simulink model "VDCHyd2022a"  (R2022a)
settings: Solver=daessc  StartTime=0.0  StopTime=simulationEndTime  FixedStep=0.001  RelTol=1e-2
values from neighbouring files (symbols this model uses):
  aux = thetaXrLB(i)    [initInertiaUpdate.m]
  Bc1_V = [0;0;0;0;0;0]    [InitializeSimulationParameters.m]
  Bc1_Vr = [0;0;0;0;0;0]    [InitializeSimulationParameters.m]
  D22Fr = [0;0;0;0;0;0]    [InitializeSimulationParameters.m]
  filtDF = init2ndOrderLowPassFilter(filtDF.cutOffFrequency,1,controller.dT)    [initializeLowPassFilters.m]
  filtDV = init2ndOrderLowPassFilter(filtDV.cutOffFrequency,1,controller.dT)    [initializeLowPassFilters.m]
  filtEnc = init2ndOrderLowPassFilter(filtEnc.cutOffFrequency,1,controller.dT)    [initializeLowPassFilters.m]
  filtPres = init2ndOrderLowPassFilter(filtPres.cutOffFrequency,1,controller.dT)    [initializeLowPassFilters.m]
  MODE = 1    [RUN_ME.m]
  s = tf('s')    [init2ndOrderLowPassFilter.m]
undefined symbols (not defined in the file or in its folder): B11_r_B11Tc1, B11_V, B11_Vr, B11Ftot_r, B12_r_B12Tc2, B12_Rot_Tc2, B12_U_Tc2, B12_V, B12_Vr, B12Ftot_r, B31_r_B31B41, B31_V, B31_Vr, B31FTot_r, B32_r_B32B42, B32_Rot_B42, B32_U_B42, B32_V, B32_Vr, B32FTot_r, B41_r_B41Tc1, B41_V, B41_Vr, B41FTot_r, B42_r_B42Tc2, B42_Rot_Tc2, B42_U_Tc2, B42_V, B42_Vr, B42FTot_r, B52_r_B52P32, B52_Rot_P32, B52_U_P32, B52_V, B52_Vr, B52Ftot_r, Bc1_r_Bc1B11, Bc1_r_Bc1B31, Bc1FTot_r, Bc2_r_Bc2B12, Bc2_r_Bc2B32, Bc2_Rot_B12, Bc2_Rot_B32, Bc2_U_B12, Bc2_U_B32, Bc2_V, Bc2_Vr, Bc2Tot_r, controller, cyl1, cyl2, cylT2, D22_V, D22_Vr, DiscIntNeverNeededParam, dq1, dq11, dq11r, dq12, dq12r ... (+119)
libraries: sm_lib x34, nesl_utility x15, simulink x11, dspinverses x1
(part 11 of 12)

== matlab function VDCHyd2022a/sbVDCController/sbFormTotalRequiredForces/sbTotalRequiredForcesPS2/regressorYB52r ==
  data: B52Vr input; B52dVr input; B52V input; B52_Rot_W input; gravity parameter; YB52r output
function YB52r  = inertiaRegressor(B52Vr, B52dVr, B52V, B52_Rot_W,  gravity)

    % Forms regressor matrix YB42r as described in Appendix A of
    % Zhu, Wen-Hong. Virtual decomposition control: toward hyper degrees
    % of freedom robots. Vol. 60. Springer Science & Business Media, 2010.

    % The code below is not the most apparent 1-to-1 visual mapping to the
    % book equations since it was generated using a symbolic toolbox.

    vxr = B52Vr(1); vyr = B52Vr(2); vzr = B52Vr(3);
    wxr = B52Vr(4); wyr = B52Vr(5); wzr = B52Vr(6);
    
    axr = B52dVr(1); ayr = B52dVr(2); azr = B52dVr(3);
    dwxr = B52dVr(4); dwyr = B52dVr(5); dwzr = B52dVr(6);
    
    wx = B52V(4); wy = B52V(5); wz = B52V(6);
    
    B52g = B52_Rot_W*gravity.Wg;
    
    gx = B52g(1); gy = B52g(2); gz = B52g(3);
    
    Y11 = (-vyr * wz + vzr * wy + axr + gx);
    t5 = (wy * wyr);
    t6 = (wz * wzr);
    Y12 = -t5 - t6;
    t7 = (wxr * wy);
    Y13 = (t7 - dwzr);
    t8 = (wxr * wz);
    Y14  = (t8 + dwyr);
    Y15 = 0;
    Y16 = 0;
    Y17 = 0;
    Y18  = 0;
    Y19 = 0;
    Y110 = 0;
    Y111 = 0;
    Y112 = 0;
    Y113 = 0;
    Y21 = vxr * wz - vzr * wx + ayr + gy;
    t11 = wx * wyr;
    Y22 = t11 + dwzr;
    t12 = wx * wxr;
    Y23 = -t12 - t6;
    t13 = wyr * wz;
    Y24 = t13 - dwxr;
    Y25 = 0;
    Y26 = 0;
    Y27 = 0;
    Y28 = 0;
    Y29 = 0;
    Y210 = 0;
    Y211 = 0;
    Y212 = 0;
    Y213 = 0;
    Y31 = -vxr * wy + vyr * wx + azr + gz;
    t16 = wx * wzr;
    Y32 = t16 - dwyr;
    t17 = wy * wzr;
    Y33 = t17 + dwxr;
    Y34 = -t12 - t5;
    Y35 = 0;
    Y36 = 0;
    Y37 = 0;
    Y38 = 0;
    Y39 = 0;
    Y310 = 0;
    Y311 = 0;
    Y312 = 0;
    Y313 = 0;
    Y41 = 0;
    Y42 = 0;
    Y43 = Y31;
    Y44 = -Y21;
    Y45 = 0;
    Y46 = Y33;
    Y47 = -Y24;
    Y48 = Y32;
    Y49 = -Y22;
    Y410 = -t5 + t6;
    Y411 = t17 - t13 + dwxr;
    Y412 = -t13;
    Y413 = t17;
    Y51 = 0;
    Y52 = -Y43;
    Y53 = 0;
    Y54 = Y11;
    Y55 = -Y48;
    Y56 = 0;
    Y57 = Y14;
    Y58 = -Y46;
    Y59 = t12 - t6;
    Y510 = Y13;
    Y511 = t8;
    Y512 = -t16 + Y511 + dwyr;
    Y513 = -t16;
    Y61 = 0;
    Y62 = Y21;
    Y63 = -Y54;
    Y64 = 0;
    Y65 = Y22;
    Y66 = -Y510;
    Y67 = 0;
    Y68 = -t12 + t5;
    Y69 = Y24;
    Y610 = -Y57;
    Y611 = -t7;
    Y612 = t11;
    Y613 = Y612 + Y611 + dwzr;
    
    
    YB52r = [Y11 Y12 Y13 Y14 Y15 Y16 Y17 Y18 Y19 Y110 Y111 Y112 Y113;...
             Y21 Y22 Y23 Y24 Y25 Y26 Y27 Y28 Y29 Y210 Y211 Y212 Y213;...
             Y31 Y32 Y33 Y34 Y35 Y36 Y37 Y38 Y39 Y310 Y311 Y312 Y313;...
             Y41 Y42 Y43 Y44 Y45 Y46 Y47 Y48 Y49 Y410 Y411 Y412 Y413;...
             Y51 Y52 Y53 Y54 Y55 Y56 Y57 Y58 Y59 Y510 Y511 Y512 Y513;...
             Y61 Y62 Y63 Y64 Y65 Y66 Y67 Y68 Y69 Y610 Y611 Y612 Y613];

end

== matlab function VDCHyd2022a/sbVDCController/sbFormAnalyticQuantities/sbRevoluteSegment1/sbGeomPropRS1/sbLiftPistonVelocity/liftPistonVelocity ==
  data: dq1 input; x1 input; q1 input; dx1 output; geom parameter; cyl1 parameter
function dx1 = liftPistonVelocity(dq1, x1, q1, geom, cyl1)

    % Calculates lift piston velocity per the paper equation (21).
    dx1 = -(geom.L1*geom.L11*sin(q1))/(x1+cyl1.x0)*dq1;

end

== matlab function VDCHyd2022a/sbVDCController/sbFormAnalyticQuantities/sbRevoluteSegment1/sbGeomPropRS1/sbq11AngleVelocity/q11AngleRate ==
  data: x1 input; q11 input; dx1 input; dq11 output; geom parameter; cyl1 parameter
function dq11 = q11AngleRate(x1, q11, dx1, geom, cyl1)
    
    % Calculates q11 angle rate per the paper equation (22).
    dq11 = -((x1+cyl1.x0)-geom.L1*cos(q11))/((x1+cyl1.x0)*geom.L1*sin(q11))*dx1;

end

== matlab function VDCHyd2022a/sbVDCController/sbFormAnalyticQuantities/sbRevoluteSegment1/sbGeomPropRS1/sbq12AngleRate/q12AngleRate ==
  data: x1 input; q12 input; dx1 input; dq12 output; geom parameter; cyl1 parameter
function dq12 = q12AngleRate(x1, q12, dx1, geom, cyl1)

    % Calculates q12 angle rate per the paper equation (23). 
    dq12 = -((x1+cyl1.x0)-geom.L11*cos(q12))/((x1+cyl1.x0)*geom.L11*sin(q12))*dx1;

end

== matlab function VDCHyd2022a/sbVDCController/sbFormAnalyticQuantities/sbRevoluteSegment1/sbPosVecsRS1/B31_r_B31B41 ==
  data: x1 input; B31_r_B31B41 output; posVec parameter
function B31_r_B31B41 = B31_r_B31B41(x1, posVec)

    % position vector of {B41} frame at lift piston tip w.r.t. {B31} frame at 
    % lift cylinder connection point [m]
    B31_r_B31B41 = posVec.B31_r_B31B31p + [x1;0;0];

end

== matlab function VDCHyd2022a/sbVDCController/sbFormAnalyticQuantities/sbRevoluteSegment1/sbRotMatsRS1/B41_Rot_Tc1 ==
  data: q12 input; B41_Rot_Tc1 output
function B41_Rot_Tc1 = B41_Rot_Tc1(q12)

    B41_Rot_Tc1 = [+cos(q12) -sin(q12) 0;...
                   +sin(q12) +cos(q12) 0;...
                       0        0      1];

end

== matlab function VDCHyd2022a/sbVDCController/sbFormAnalyticQuantities/sbRevoluteSegment1/sbRotMatsRS1/Bc1_Rot_B11 ==
  data: q1 input; Bc1_Rot_B11 output
function Bc1_Rot_B11 = Bc1_Rot_B11(q1)

    Bc1_Rot_B11 = [+cos(q1) -sin(q1) 0;...
                   +sin(q1) +cos(q1) 0;...
                      0        0     1];

end

== matlab function VDCHyd2022a/sbVDCController/sbFormAnalyticQuantities/sbRevoluteSegment1/sbRotMatsRS1/Bc1_Rot_B31 ==
  data: q11 input; Bc1_Rot_B31 output
function Bc1_Rot_B31 = Bc1_Rot_B31(q11)

    Bc1_Rot_B31 = [+cos(q11) -sin(q11) 0;...
                   +sin(q11) +cos(q11) 0;...
                       0         0     1];

end

== matlab function VDCHyd2022a/sbVDCController/sbFormingControlActions/regressorYdt2 ==
  data: dfpt2r input; Ydt2 output; xt2 input; dxt2 input; pat2 input; pbt2 input; hosingT2 parameter; cylT2 parameter
function Ydt2 = cylinderRegressor(dfpt2r, xt2, dxt2, pat2, pbt2, hosingT2, cylT2)

    %Implemented per (43) in S. Lampinen, J. Koivumäki and J. Mattila, 
    % "Improved Hydraulic Cylinder Model for the Virtual Decomposition 
    % Control Approach," 2019 IEEE International Conference on Cybernetics 
    % and Intelligent Systems (CIS) and IEEE Conference on Robotics, 
    % Automation and Mechatronics (RAM), Bangkok, Thailand, 2019, 
    % pp. 113-118, doi: 10.1109/CIS-RAM47153.2019.9095788.
    Ydt2 = [dfpt2r,...
            dxt2/(hosingT2.V0a/cylT2.Aa + xt2),...
            dxt2/(hosingT2.V0b/cylT2.Ab + cylT2.sp - xt2),...
            ((pat2-pbt2)*(cylT2.Aa*hosingT2.V0b + cylT2.Ab*hosingT2.V0a + cylT2.Aa*cylT2.Ab*cylT2.sp))/((hosingT2.V0a + cylT2.Aa*xt2)*(hosingT2.V0b + cylT2.Ab*(cylT2.sp - xt2)))];

end

== matlab function VDCHyd2022a/sbVDCController/sbFormAnalyticQuantities/sbRevoluteSegment1/sbUMatsRS1/B11_U_Tc1 ==
  data: B11_r_B11Tc1 input; B11_U_Tc1 output; B11_Rot_Tc1 input
function B11_U_Tc1 = B11_U_Tc1(B11_r_B11Tc1, B11_Rot_Tc1)

     % Velocity/force transformation matrix per equation (5).
    B11_U_Tc1 = [B11_Rot_Tc1,                    zeros(3);...
                 dual(B11_r_B11Tc1)*B11_Rot_Tc1, B11_Rot_Tc1];
   
end
   
function dual_r = dual(ArAB)

    % Skew-symmetric operator as defined by equation (6).
    dual_r = [0,  -ArAB(3), ArAB(2);...
              ArAB(3), 0, -ArAB(1);...
              -ArAB(2), ArAB(1), 0];

end

== matlab function VDCHyd2022a/sbVDCController/sbFormAnalyticQuantities/sbRevoluteSegment1/sbUMatsRS1/B31_U_B41 ==
  data: B31_r_B31B41 input; B31_U_B41 output; B31_Rot_B41 input
function B31_U_B41 = B31_U_B41(B31_r_B31B41, B31_Rot_B41)

    % Velocity/force transformation matrix per equation (5).
    B31_U_B41 = [B31_Rot_B41,                    zeros(3);...
                 dual(B31_r_B31B41)*B31_Rot_B41, B31_Rot_B41];
   
end
   
function dual_r = dual(ArAB)

     % Skew-symmetric operator as defined by equation (6). 
    dual_r = [0,  -ArAB(3), ArAB(2);...
              ArAB(3), 0, -ArAB(1);...
              -ArAB(2), ArAB(1), 0];

end

== matlab function VDCHyd2022a/sbVDCController/sbFormAnalyticQuantities/sbRevoluteSegment1/sbUMatsRS1/B41_U_Tc1 ==
  data: B41_r_B41Tc1 input; B41_U_Tc1 output; B41_Rot_Tc1 input
function B41_U_Tc1 = B41_U_Tc1(B41_r_B41Tc1, B41_Rot_Tc1)

    % Velocity/force transformation matrix per equation (5).
    B41_U_Tc1 = [B41_Rot_Tc1,                    zeros(3);...
                 dual(B41_r_B41Tc1)*B41_Rot_Tc1, B41_Rot_Tc1];
   
end
   
function dual_r = dual(ArAB)

    % Skew-symmetric operator as defined by equation (6).
    dual_r = [0,  -ArAB(3), ArAB(2);...
              ArAB(3), 0, -ArAB(1);...
              -ArAB(2), ArAB(1), 0];

end

== matlab function VDCHyd2022a/sbVDCController/sbFormAnalyticQuantities/sbRevoluteSegment1/sbUMatsRS1/Bc1_U_B11 ==
  data: Bc1_r_Bc1B11 input; Bc1_U_B11 output; Bc1_Rot_B11 input
function Bc1_U_B11 = Bc1_U_B11(Bc1_r_Bc1B11, Bc1_Rot_B11)

    % Velocity/force transformation matrix per equation (5).
    Bc1_U_B11 = [Bc1_Rot_B11,                    zeros(3);...
                 dual(Bc1_r_Bc1B11)*Bc1_Rot_B11, Bc1_Rot_B11];
   
end
   
function dual_r = dual(ArAB)

    % Skew-symmetric operator as defined by equation (6).
    dual_r = [0,  -ArAB(3), ArAB(2);...
              ArAB(3), 0, -ArAB(1);...
              -ArAB(2), ArAB(1), 0];

end

== matlab function VDCHyd2022a/sbVDCController/sbFormAnalyticQuantities/sbRevoluteSegment1/sbUMatsRS1/Bc1_U_B31 ==
  data: Bc1_r_Bc1B31 input; Bc1_U_B31 output; Bc1_Rot_B31 input
function Bc1_U_B31 = Bc1_U_B31(Bc1_r_Bc1B31, Bc1_Rot_B31)

    % Velocity/force transformation matrix per equation (5).
    Bc1_U_B31 = [Bc1_Rot_B31,                    zeros(3);...
                 dual(Bc1_r_Bc1B31)*Bc1_Rot_B31, Bc1_Rot_B31];
   
end
   
function dual_r = dual(ArAB)

    
    % Skew-symmetric operator as defined by equation (6). 
    dual_r = [0,  -ArAB(3), ArAB(2);...
              ArAB(3), 0, -ArAB(1);...
              -ArAB(2), ArAB(1), 0];

end

== matlab function VDCHyd2022a/sbVDCController/sbFormAnalyticQuantities/sbRevoluteSegment1/sbUMatsRS1/Tc1_U_Bc2 ==
  data: Tc1_r_Tc1Bc2 input; Tc1_U_Bc2 output; Tc1_Rot_Bc2 input
function Tc1_U_Bc2 = Tc1_U_Bc2(Tc1_r_Tc1Bc2, Tc1_Rot_Bc2)

    % Velocity/force transformation matrix per equation (5).
    Tc1_U_Bc2 = [Tc1_Rot_Bc2,                    zeros(3);...
                 dual(Tc1_r_Tc1Bc2)*Tc1_Rot_Bc2, Tc1_Rot_Bc2];
   
end
   
function dual_r = dual(ArAB)

    % Skew-symmetric operator as defined by equation (6).   
    dual_r = [0,  -ArAB(3), ArAB(2);...
              ArAB(3), 0, -ArAB(1);...
              -ArAB(2), ArAB(1), 0];

end

== matlab function VDCHyd2022a/sbVDCController/sbFormAnalyticQuantities/sbPrismaticSegment2/sbPosVecsPS2/P22_r_P22B52 ==
  data: xt2 input; P22_r_P22B52 output; posVec parameter
function P22_r_P22B52 = P22_r_P22B52(xt2, posVec)

    % position vector of {B52} frame at the extension piston tip w.r.t.
    % {P22} frame at extension cylinder connection point [m]
    P22_r_P22B52 = posVec.P22_r_P22P22p + [xt2; 0; 0];

end

== matlab function VDCHyd2022a/sbVDCController/sbFormAnalyticQuantities/sbPrismaticSegment2/sbUMatsPS2/B52_U_P32 ==
  data: B52_r_B52B32 input; B52_U_P32 output; B52_Rot_B32 input
function B52_U_P32 = B52_U_P32(B52_r_B52B32, B52_Rot_B32)

    % Velocity/force transformation matrix per equation (5).
    B52_U_P32 = [B52_Rot_B32,                    zeros(3);...
                 dual(B52_r_B52B32)*B52_Rot_B32, B52_Rot_B32];
   
end
   
function dual_r = dual(ArAB)

    % Skew-symmetric operator as defined by equation (6)
    dual_r = [0,  -ArAB(3), ArAB(2);...
              ArAB(3), 0, -ArAB(1);...
              -ArAB(2), ArAB(1), 0];

end

== matlab function VDCHyd2022a/sbVDCController/sbFormAnalyticQuantities/sbPrismaticSegment2/sbUMatsPS2/P22_U_B52 ==
  data: P22_r_P22B52 input; P22_U_B52 output; P22_Rot_B52 input
function P22_U_B52 = P22_U_B52(P22_r_P22B52, P22_Rot_B52)

    % Velocity/force transformation matrix per equation (5).
    P22_U_B52 = [P22_Rot_B52,                    zeros(3);...
                 dual(P22_r_P22B52)*P22_Rot_B52, P22_Rot_B52];
   
end
   
function dual_r = dual(ArAB)

    % Skew-symmetric operator as defined by equation (6).
    dual_r = [0,  -ArAB(3), ArAB(2);...
              ArAB(3), 0, -ArAB(1);...
              -ArAB(2), ArAB(1), 0];

end

== matlab function VDCHyd2022a/sbVDCController/sbFormAnalyticQuantities/sbPrismaticSegment2/sbUMatsPS2/P32_U_D22 ==
  data: P32_r_P32D22 input; P32_U_D22 output; P32_Rot_D22 input
function P32_U_D22 = P32_U_D22(P32_r_P32D22, P32_Rot_D22)

    % Velocity/force transformation matrix per equation (5).
    P32_U_D22 = [P32_Rot_D22,                    zeros(3);...
                  dual(P32_r_P32D22)*P32_Rot_D22, P32_Rot_D22];
   
end
   
function dual_r = dual(ArAB)

    % Skew-symmetric operator as defined by equation (6)
    dual_r = [0,  -ArAB(3), ArAB(2);...
              ArAB(3), 0, -ArAB(1);...
              -ArAB(2), ArAB(1), 0];

end

== matlab function VDCHyd2022a/sbVDCController/sbFormAnalyticQuantities/sbRevoluteSegment2/sbPosVecsRS2/B32_r_B32B42 ==
  data: x2 input; B32_r_B32B42 output; posVec parameter
function B32_r_B32B42 = B32_r_B32B42(x2, posVec)

    B32_r_B32B42 = posVec.B32_r_B32B32p + [x2;0;0];

end

== matlab function VDCHyd2022a/sbVDCController/sbFormAnalyticQuantities/sbRevoluteSegment2/sbRotMatsRS2/B42_Rot_Tc2 ==
  data: q22 input; B42_Rot_Tc2 output
function B42_Rot_Tc2 = B42_Rot_Tc2(q22)

    B42_Rot_Tc2 = [+cos(q22) -sin(q22) 0;...
                   +sin(q22) +cos(q22) 0;...
                       0        0      1];

end

== matlab function VDCHyd2022a/sbVDCController/sbFormAnalyticQuantities/sbRevoluteSegment2/sbRotMatsRS2/Bc2_Rot_B12 ==
  data: q2 input; Bc2_Rot_B12 output
function Bc2_Rot_B12 = Bc2_Rot_B12(q2)

    Bc2_Rot_B12 = [+cos(q2) -sin(q2) 0;...
                   +sin(q2) +cos(q2) 0;...
                      0        0     1];

end

== matlab function VDCHyd2022a/sbVDCController/sbFormAnalyticQuantities/sbRevoluteSegment2/sbRotMatsRS2/Bc2_Rot_B32 ==
  data: q21 input; Bc2_Rot_B32 output
function Bc2_Rot_B32 = Bc2_Rot_B32(q21)

    Bc2_Rot_B32 = [+cos(q21) -sin(q21) 0;...
                   +sin(q21) +cos(q21) 0;...
                       0         0     1];

end

== matlab function VDCHyd2022a/sbVDCController/sbFormAnalyticQuantities/sbRevoluteSegment2/sbUMatsRS2/B12_U_Tc2 ==
  data: B12_r_B12Tc2 input; B12_U_Tc2 output; B12_Rot_Tc2 input
function B12_U_Tc2 = B12_U_Tc2(B12_r_B12Tc2, B12_Rot_Tc2)

    % Velocity/force transformation matrix per equation (5).
    B12_U_Tc2 = [B12_Rot_Tc2,                    zeros(3);...
                 dual(B12_r_B12Tc2)*B12_Rot_Tc2, B12_Rot_Tc2];
   
end
   
function dual_r = dual(ArAB)

    % Skew-symmetric operator as defined by equation (6).
    dual_r = [0,  -ArAB(3), ArAB(2);...
              ArAB(3), 0, -ArAB(1);...
              -ArAB(2), ArAB(1), 0];

end

== matlab function VDCHyd2022a/sbVDCController/sbFormAnalyticQuantities/sbRevoluteSegment2/sbUMatsRS2/B32_U_B42 ==
  data: B32_r_B32B42 input; B32_U_B42 output; B32_Rot_B42 input
function B32_U_B42 = B32_U_B42(B32_r_B32B42, B32_Rot_B42)

    % Velocity/force transformation matrix per equation (5).
    B32_U_B42 = [B32_Rot_B42,                    zeros(3);...
                 dual(B32_r_B32B42)*B32_Rot_B42, B32_Rot_B42];
   
end
   
function dual_r = dual(ArAB)

    % Skew-symmetric operator as defined by equation (6).
    dual_r = [0,  -ArAB(3), ArAB(2);...
              ArAB(3), 0, -ArAB(1);...
              -ArAB(2), ArAB(1), 0];

end

== matlab function VDCHyd2022a/sbVDCController/sbFormingControlActions/regressorYv2 ==
  data: u2 input; Yv2 output; pS input; pR input; pa2 input; pb2 input; x2 input; hosing2 parameter; cyl2 parameter
function Yv2 = valveRegressor(u2, pS, pR, pa2, pb2, x2, hosing2, cyl2)

    % Implemented per (25) in S. Lampinen, J. Koivumäki and J. Mattila, 
    % "Improved Hydraulic Cylinder Model for the Virtual Decomposition 
    % Control Approach," 2019 IEEE International Conference on Cybernetics 
    % and Intelligent Systems (CIS) and IEEE Conference on Robotics, 
    % Automation and Mechatronics (RAM), Bangkok, Thailand, 2019, 
    % pp. 113-118, doi: 10.1109/CIS-RAM47153.2019.9095788 in order
    % Yv = [cp1, cn1, cp2, cn2]
    Yv2 = [sqAbsPresDrop(pS - pa2)*selFcn(u2)*u2/(hosing2.V0a/cyl2.Aa + x2),...
           sqAbsPresDrop(pa2 - pR)*selFcn(-u2)*u2/(hosing2.V0a/cyl2.Aa + x2),...
           sqAbsPresDrop(pS - pb2)*selFcn(-u2)*u2/(hosing2.V0b/cyl2.Ab + cyl2.sp - x2),...
           sqAbsPresDrop(pb2 - pR)*selFcn(u2)*u2/(hosing2.V0b/cyl2.Ab + cyl2.sp - x2)];

end

function S = selFcn(U)

    if U > 0
        S = 1;
    else
        S = 0;
    end
    
end

function nup = sqAbsPresDrop(dp)

    nup = sign(dp)*sqrt(abs(dp));

end

== matlab function VDCHyd2022a/sbVDCController/sbFormAnalyticQuantities/sbRevoluteSegment2/sbUMatsRS2/B42_U_Tc2 ==
  data: B42_r_B42Tc2 input; B42_U_Tc2 output; B42_Rot_Tc2 input
function B42_U_Tc2 = B42_U_Tc2(B42_r_B42Tc2, B42_Rot_Tc2)

    % Velocity/force transformation matrix per equation (5).
    B42_U_Tc2 = [B42_Rot_Tc2,                    zeros(3);...
                 dual(B42_r_B42Tc2)*B42_Rot_Tc2, B42_Rot_Tc2];
   
end
   
function dual_r = dual(ArAB)

    % Skew-symmetric operator as defined by equation (6).
    dual_r = [0,  -ArAB(3), ArAB(2);...
              ArAB(3), 0, -ArAB(1);...
              -ArAB(2), ArAB(1), 0];

end

== matlab function VDCHyd2022a/sbVDCController/sbFormAnalyticQuantities/sbRevoluteSegment2/sbUMatsRS2/Bc2_U_B12 ==
  data: Bc2_r_Bc2B12 input; Bc2_U_B12 output; Bc2_Rot_B12 input
function Bc2_U_B12 = Bc2_U_B12(Bc2_r_Bc2B12, Bc2_Rot_B12)

    % Velocity/force transformation matrix per equation (5).
    Bc2_U_B12 = [Bc2_Rot_B12,                    zeros(3);...
                 dual(Bc2_r_Bc2B12)*Bc2_Rot_B12, Bc2_Rot_B12];
   
end
   
function dual_r = dual(ArAB)

    % Skew-symmetric operator as defined by equation (6).
    dual_r = [0,  -ArAB(3), ArAB(2);...
              ArAB(3), 0, -ArAB(1);...
              -ArAB(2), ArAB(1), 0];

end

== matlab function VDCHyd2022a/sbVDCController/sbFormAnalyticQuantities/sbRevoluteSegment2/sbUMatsRS2/Bc2_U_B32 ==
  data: Bc2_r_Bc2B32 input; Bc2_U_B32 output; Bc2_Rot_B32 input
function Bc2_U_B32 = Bc2_U_B32(Bc2_r_Bc2B32, Bc2_Rot_B32)
    
    % Velocity/force transformation matrix per equation (5).
    Bc2_U_B32 = [Bc2_Rot_B32,                    zeros(3);...
             dual(Bc2_r_Bc2B32)*Bc2_Rot_B32, Bc2_Rot_B32];
   
end
   
function dual_r = dual(ArAB)

    % Skew-symmetric operator as defined by equation (6).
    dual_r = [0,  -ArAB(3), ArAB(2);...
              ArAB(3), 0, -ArAB(1);...
              -ArAB(2), ArAB(1), 0];

end

== matlab function VDCHyd2022a/sbVDCController/sbFormAnalyticQuantities/sbRevoluteSegment2/sbUMatsRS2/Tc2_U_P22 ==
  data: Tc2_r_Tc2P22 input; Tc2_U_P22 output; Tc2_Rot_P22 input
function Tc2_U_P22 = Tc2_U_P22(Tc2_r_Tc2P22, Tc2_Rot_P22)

    % Velocity/force transformation matrix per equation (5).
    Tc2_U_P22 = [Tc2_Rot_P22,                    zeros(3);...
                 dual(Tc2_r_Tc2P22)*Tc2_Rot_P22, Tc2_Rot_P22];
   
end
   
function dual_r = dual(ArAB)
    
    % Skew-symmetric operator as defined by equation (6).
    dual_r = [0,  -ArAB(3), ArAB(2);...
              ArAB(3), 0, -ArAB(1);...
              -ArAB(2), ArAB(1), 0];

end

== matlab function VDCHyd2022a/sbVDCController/sbFormAnalyticQuantities/sbRevoluteSegment1/sbGeomPropRS1req/sbRequiredLiftPistonVelocity/requiredLiftPistonVelocity ==
  data: dq1r input; x1 input; q1 input; dx1r output; geom parameter; cyl1 parameter
function dx1r = requiredLiftPistonVelocity(dq1r, x1, q1, geom, cyl1)

    % calculates required lift piston velocity relying on the paper equation (21).
    dx1r = -(geom.L1*geom.L11*sin(q1))/(x1+cyl1.x0)*dq1r;

end

== matlab function VDCHyd2022a/sbVDCController/sbFormAnalyticQuantities/sbRevoluteSegment1/sbGeomPropRS1req/sbRequiredq11AngleRate/requiredq11AngleRate ==
  data: x1 input; q11 input; dx1r input; dq11r output; geom parameter; cyl1 parameter
function dq11r = requiredq11AngleRate(x1, q11, dx1r, geom, cyl1)

    % Calculate the required q11 angle rate relying on the paper equation (22).
    dq11r = -((x1+cyl1.x0)-geom.L1*cos(q11))/((x1+cyl1.x0)*geom.L1*sin(q11))*dx1r;

end

== matlab function VDCHyd2022a/sbVDCController/sbFormAnalyticQuantities/sbRevoluteSegment1/sbGeomPropRS1req/sbRequiredq12AngleRate/requiredq12AngleRate ==
  data: x1 input; q12 input; dx1r input; dq12r output; geom parameter; cyl1 parameter
function dq12r = requiredq12AngleRate(x1, q12, dx1r, geom, cyl1)

    % Calculates the required q12 angle rate relying on the paper equation (23).
    dq12r = -((x1+cyl1.x0)-geom.L11*cos(q12))/((x1+cyl1.x0)*geom.L11*sin(q12))*dx1r;

end

== matlab function VDCHyd2022a/sbVDCController/sbFormingControlActions/regressorYv1 ==
  data: u1 input; Yv1 output; pS input; pR input; pa1 input; pb1 input; x1 input; hosing1 parameter; cyl1 parameter
function Yv1 = valveRegressor(u1, pS, pR, pa1, pb1, x1, hosing1, cyl1)

    
    % Implemented per (25) in S. Lampinen, J. Koivumäki and J. Mattila, 
    % "Improved Hydraulic Cylinder Model for the Virtual Decomposition 
    % Control Approach," 2019 IEEE International Conference on Cybernetics 
    % and Intelligent Systems (CIS) and IEEE Conference on Robotics, 
    % Automation and Mechatronics (RAM), Bangkok, Thailand, 2019, 
    % pp. 113-118, doi: 10.1109/CIS-RAM47153.2019.9095788 in order
    % Yv = [cp1, cn1, cp2, cn2]
    Yv1 = [sqAbsPresDrop(pS - pa1)*selFcn(u1)*u1/(hosing1.V0a/cyl1.Aa + x1),...
           sqAbsPresDrop(pa1 - pR)*selFcn(-u1)*u1/(hosing1.V0a/cyl1.Aa + x1),...
           sqAbsPresDrop(pS - pb1)*selFcn(-u1)*u1/(hosing1.V0b/cyl1.Ab + cyl1.sp - x1),...
           sqAbsPresDrop(pb1 - pR)*selFcn(u1)*u1/(hosing1.V0b/cyl1.Ab + cyl1.sp - x1)];

end

function S = selFcn(U)

    if U > 0
        S = 1;
    else
        S = 0;
    end
    
end

function nup = sqAbsPresDrop(dp)

    nup = sign(dp)*sqrt(abs(dp));

end

== matlab function VDCHyd2022a/sbVDCController/sbFormTotalRequiredForces/sbTotalRequiredForcesPS2/regressorYP22r ==
  data: P22Vr input; P22dVr input; P22V input; P22_Rot_W input; gravity parameter; YP22r output
function YP22r  = inertiaRegressor(P22Vr, P22dVr, P22V, P22_Rot_W,  gravity)

    % Forms regressor matrix YB42r as described in Appendix A of
    % Zhu, Wen-Hong. Virtual decomposition control: toward hyper degrees
    % of freedom robots. Vol. 60. Springer Science & Business Media, 2010.

    % The code below is not the most apparent 1-to-1 visual mapping to the
    % book equations since it was generated using a symbolic toolbox.

    vxr = P22Vr(1); vyr = P22Vr(2); vzr = P22Vr(3);
    wxr = P22Vr(4); wyr = P22Vr(5); wzr = P22Vr(6);
    
    axr = P22dVr(1); ayr = P22dVr(2); azr = P22dVr(3);
    dwxr = P22dVr(4); dwyr = P22dVr(5); dwzr = P22dVr(6);
    
    wx = P22V(4); wy = P22V(5); wz = P22V(6);
    
    P22g = P22_Rot_W*gravity.Wg;
    
    gx = P22g(1); gy = P22g(2); gz = P22g(3);
    
    Y11 = (-vyr * wz + vzr * wy + axr + gx);
    t5 = (wy * wyr);
    t6 = (wz * wzr);
    Y12 = -t5 - t6;
    t7 = (wxr * wy);
    Y13 = (t7 - dwzr);
    t8 = (wxr * wz);
    Y14  = (t8 + dwyr);
    Y15 = 0;
    Y16 = 0;
    Y17 = 0;
    Y18  = 0;
    Y19 = 0;
    Y110 = 0;
    Y111 = 0;
    Y112 = 0;
    Y113 = 0;
    Y21 = vxr * wz - vzr * wx + ayr + gy;
    t11 = wx * wyr;
    Y22 = t11 + dwzr;
    t12 = wx * wxr;
    Y23 = -t12 - t6;
    t13 = wyr * wz;
    Y24 = t13 - dwxr;
    Y25 = 0;
    Y26 = 0;
    Y27 = 0;
    Y28 = 0;
    Y29 = 0;
    Y210 = 0;
    Y211 = 0;
    Y212 = 0;
    Y213 = 0;
    Y31 = -vxr * wy + vyr * wx + azr + gz;
    t16 = wx * wzr;
    Y32 = t16 - dwyr;
    t17 = wy * wzr;
    Y33 = t17 + dwxr;
    Y34 = -t12 - t5;
    Y35 = 0;
    Y36 = 0;
    Y37 = 0;
    Y38 = 0;
    Y39 = 0;
    Y310 = 0;
    Y311 = 0;
    Y312 = 0;
    Y313 = 0;
    Y41 = 0;
    Y42 = 0;
    Y43 = Y31;
    Y44 = -Y21;
    Y45 = 0;
    Y46 = Y33;
    Y47 = -Y24;
    Y48 = Y32;
    Y49 = -Y22;
    Y410 = -t5 + t6;
    Y411 = t17 - t13 + dwxr;
    Y412 = -t13;
    Y413 = t17;
    Y51 = 0;
    Y52 = -Y43;
    Y53 = 0;
    Y54 = Y11;
    Y55 = -Y48;
    Y56 = 0;
    Y57 = Y14;
    Y58 = -Y46;
    Y59 = t12 - t6;
    Y510 = Y13;
    Y511 = t8;
    Y512 = -t16 + Y511 + dwyr;
    Y513 = -t16;
    Y61 = 0;
    Y62 = Y21;
    Y63 = -Y54;
    Y64 = 0;
    Y65 = Y22;
    Y66 = -Y510;
    Y67 = 0;
    Y68 = -t12 + t5;
    Y69 = Y24;
    Y610 = -Y57;
    Y611 = -t7;
    Y612 = t11;
    Y613 = Y612 + Y611 + dwzr;
    
    
    YP22r = [Y11 Y12 Y13 Y14 Y15 Y16 Y17 Y18 Y19 Y110 Y111 Y112 Y113;...
             Y21 Y22 Y23 Y24 Y25 Y26 Y27 Y28 Y29 Y210 Y211 Y212 Y213;...
             Y31 Y32 Y33 Y34 Y35 Y36 Y37 Y38 Y39 Y310 Y311 Y312 Y313;...
             Y41 Y42 Y43 Y44 Y45 Y46 Y47 Y48 Y49 Y410 Y411 Y412 Y413;...
             Y51 Y52 Y53 Y54 Y55 Y56 Y57 Y58 Y59 Y510 Y511 Y512 Y513;...
             Y61 Y62 Y63 Y64 Y65 Y66 Y67 Y68 Y69 Y610 Y611 Y612 Y613];

end

== matlab function VDCHyd2022a/sbVDCController/sbFormTotalRequiredForces/sbTotalRequiredForcesPS2/regressorYP32r ==
  data: P32Vr input; P32dVr input; P32V input; P32_Rot_W input; gravity parameter; YP32r output
function YP32r  = inertiaRegressor(P32Vr, P32dVr, P32V, P32_Rot_W,  gravity)
    
    % Forms regressor matrix YB42r as described in Appendix A of
    % Zhu, Wen-Hong. Virtual decomposition control: toward hyper degrees
    % of freedom robots. Vol. 60. Springer Science & Business Media, 2010.

    % The code below is not the most apparent 1-to-1 visual mapping to the
    % book equations since it was generated using a symbolic toolbox.

    vxr = P32Vr(1); vyr = P32Vr(2); vzr = P32Vr(3);
    wxr = P32Vr(4); wyr = P32Vr(5); wzr = P32Vr(6);
    
    axr = P32dVr(1); ayr = P32dVr(2); azr = P32dVr(3);
    dwxr = P32dVr(4); dwyr = P32dVr(5); dwzr = P32dVr(6);
    
    wx = P32V(4); wy = P32V(5); wz = P32V(6);
    
    P32g = P32_Rot_W*gravity.Wg;
    
    gx = P32g(1); gy = P32g(2); gz = P32g(3);
    
    Y11 = (-vyr * wz + vzr * wy + axr + gx);
    t5 = (wy * wyr);
    t6 = (wz * wzr);
    Y12 = -t5 - t6;
    t7 = (wxr * wy);
    Y13 = (t7 - dwzr);
    t8 = (wxr * wz);
    Y14  = (t8 + dwyr);
    Y15 = 0;
    Y16 = 0;
    Y17 = 0;
    Y18  = 0;
    Y19 = 0;
    Y110 = 0;
    Y111 = 0;
    Y112 = 0;
    Y113 = 0;
    Y21 = vxr * wz - vzr * wx + ayr + gy;
    t11 = wx * wyr;
    Y22 = t11 + dwzr;
    t12 = wx * wxr;
    Y23 = -t12 - t6;
    t13 = wyr * wz;
    Y24 = t13 - dwxr;
    Y25 = 0;
    Y26 = 0;
    Y27 = 0;
    Y28 = 0;
    Y29 = 0;
    Y210 = 0;
    Y211 = 0;
    Y212 = 0;
    Y213 = 0;
    Y31 = -vxr * wy + vyr * wx + azr + gz;
    t16 = wx * wzr;
    Y32 = t16 - dwyr;
    t17 = wy * wzr;
    Y33 = t17 + dwxr;
    Y34 = -t12 - t5;
    Y35 = 0;
    Y36 = 0;
    Y37 = 0;
    Y38 = 0;
    Y39 = 0;
    Y310 = 0;
    Y311 = 0;
    Y312 = 0;
    Y313 = 0;
    Y41 = 0;
    Y42 = 0;
    Y43 = Y31;
    Y44 = -Y21;
    Y45 = 0;
    Y46 = Y33;
    Y47 = -Y24;
    Y48 = Y32;
    Y49 = -Y22;
    Y410 = -t5 + t6;
    Y411 = t17 - t13 + dwxr;
    Y412 = -t13;
    Y413 = t17;
    Y51 = 0;
    Y52 = -Y43;
    Y53 = 0;
    Y54 = Y11;
    Y55 = -Y48;
    Y56 = 0;
    Y57 = Y14;
    Y58 = -Y46;
    Y59 = t12 - t6;
    Y510 = Y13;
    Y511 = t8;
    Y512 = -t16 + Y511 + dwyr;
    Y513 = -t16;
    Y61 = 0;
    Y62 = Y21;
    Y63 = -Y54;
    Y64 = 0;
    Y65 = Y22;
    Y66 = -Y510;
    Y67 = 0;
    Y68 = -t12 + t5;
    Y69 = Y24;
    Y610 = -Y57;
    Y611 = -t7;
    Y612 = t11;
    Y613 = Y612 + Y611 + dwzr;
    
    
    YP32r = [Y11 Y12 Y13 Y14 Y15 Y16 Y17 Y18 Y19 Y110 Y111 Y112 Y113;...
         Y21 Y22 Y23 Y24 Y25 Y26 Y27 Y28 Y29 Y210 Y211 Y212 Y213;...
         Y31 Y32 Y33 Y34 Y35 Y36 Y37 Y38 Y39 Y310 Y311 Y312 Y313;...
         Y41 Y42 Y43 Y44 Y45 Y46 Y47 Y48 Y49 Y410 Y411 Y412 Y413;...
         Y51 Y52 Y53 Y54 Y55 Y56 Y57 Y58 Y59 Y510 Y511 Y512 Y513;...
         Y61 Y62 Y63 Y64 Y65 Y66 Y67 Y68 Y69 Y610 Y611 Y612 Y613];

end

== matlab function VDCHyd2022a/sbVDCController/sbFormTotalRequiredForces/sbTotalRequiredForcesRS2/regressorYB12r ==
  data: B12Vr input; B12dVr input; B12V input; B12_Rot_W input; gravity parameter; YB12r output
function YB12r  = inertiaRegressor(B12Vr, B12dVr, B12V, B12_Rot_W,  gravity)

    % Forms regressor matrix YB12r as described in Appendix A of
    % Zhu, Wen-Hong. Virtual decomposition control: toward hyper degrees
    % of freedom robots. Vol. 60. Springer Science & Business Media, 2010.

    % The code below is not the most apparent 1-to-1 visual mapping to the
    % book equations since it was generated using a symbolic toolbox.

    vxr = B12Vr(1); vyr = B12Vr(2); vzr = B12Vr(3);
    wxr = B12Vr(4); wyr = B12Vr(5); wzr = B12Vr(6);
    
    axr = B12dVr(1); ayr = B12dVr(2); azr = B12dVr(3);
    dwxr = B12dVr(4); dwyr = B12dVr(5); dwzr = B12dVr(6);
    
    wx = B12V(4); wy = B12V(5); wz = B12V(6);
    
    B12g = B12_Rot_W*gravity.Wg;
    
    gx = B12g(1); gy = B12g(2); gz = B12g(3);
    
    Y11 = (-vyr * wz + vzr * wy + axr + gx);
    t5 = (wy * wyr);
    t6 = (wz * wzr);
    Y12 = -t5 - t6;
    t7 = (wxr * wy);
    Y13 = (t7 - dwzr);
    t8 = (wxr * wz);
    Y14  = (t8 + dwyr);
    Y15 = 0;
    Y16 = 0;
    Y17 = 0;
    Y18  = 0;
    Y19 = 0;
    Y110 = 0;
    Y111 = 0;
    Y112 = 0;
    Y113 = 0;
    Y21 = vxr * wz - vzr * wx + ayr + gy;
    t11 = wx * wyr;
    Y22 = t11 + dwzr;
    t12 = wx * wxr;
    Y23 = -t12 - t6;
    t13 = wyr * wz;
    Y24 = t13 - dwxr;
    Y25 = 0;
    Y26 = 0;
    Y27 = 0;
    Y28 = 0;
    Y29 = 0;
    Y210 = 0;
    Y211 = 0;
    Y212 = 0;
    Y213 = 0;
    Y31 = -vxr * wy + vyr * wx + azr + gz;
    t16 = wx * wzr;
    Y32 = t16 - dwyr;
    t17 = wy * wzr;
    Y33 = t17 + dwxr;
    Y34 = -t12 - t5;
    Y35 = 0;
    Y36 = 0;
    Y37 = 0;
    Y38 = 0;
    Y39 = 0;
    Y310 = 0;
    Y311 = 0;
    Y312 = 0;
    Y313 = 0;
    Y41 = 0;
    Y42 = 0;
    Y43 = Y31;
    Y44 = -Y21;
    Y45 = 0;
    Y46 = Y33;
    Y47 = -Y24;
    Y48 = Y32;
    Y49 = -Y22;
    Y410 = -t5 + t6;
    Y411 = t17 - t13 + dwxr;
    Y412 = -t13;
    Y413 = t17;
    Y51 = 0;
    Y52 = -Y43;
    Y53 = 0;
    Y54 = Y11;
    Y55 = -Y48;
    Y56 = 0;
    Y57 = Y14;
    Y58 = -Y46;
    Y59 = t12 - t6;
    Y510 = Y13;
    Y511 = t8;
    Y512 = -t16 + Y511 + dwyr;
    Y513 = -t16;
    Y61 = 0;
    Y62 = Y21;
    Y63 = -Y54;
    Y64 = 0;
    Y65 = Y22;
    Y66 = -Y510;
    Y67 = 0;
    Y68 = -t12 + t5;
    Y69 = Y24;
    Y610 = -Y57;
    Y611 = -t7;
    Y612 = t11;
    Y613 = Y612 + Y611 + dwzr;
    
    
    YB12r = [Y11 Y12 Y13 Y14 Y15 Y16 Y17 Y18 Y19 Y110 Y111 Y112 Y113;...
    	     Y21 Y22 Y23 Y24 Y25 Y26 Y27 Y28 Y29 Y210 Y211 Y212 Y213;...
             Y31 Y32 Y33 Y34 Y35 Y36 Y37 Y38 Y39 Y310 Y311 Y312 Y313;...
             Y41 Y42 Y43 Y44 Y45 Y46 Y47 Y48 Y49 Y410 Y411 Y412 Y413;...
             Y51 Y52 Y53 Y54 Y55 Y56 Y57 Y58 Y59 Y510 Y511 Y512 Y513;...
             Y61 Y62 Y63 Y64 Y65 Y66 Y67 Y68 Y69 Y610 Y611 Y612 Y613];

end

== matlab function VDCHyd2022a/sbVDCController/sbFormTotalRequiredForces/sbTotalRequiredForcesRS2/regressorYB32r ==
  data: B32Vr input; B32dVr input; B32V input; B32_Rot_W input; gravity parameter; YB32r output
function YB32r  = YB32r( B32Vr, B32dVr, B32V, B32_Rot_W,  gravity)

    % Forms regressor matrix YB32r as described in Appendix A of
    % Zhu, Wen-Hong. Virtual decomposition control: toward hyper degrees
    % of freedom robots. Vol. 60. Springer Science & Business Media, 2010.

    % The code below is not the most apparent 1-to-1 visual mapping to the
    % book equations since it was generated using a symbolic toolbox.

    vxr = B32Vr(1); vyr = B32Vr(2); vzr = B32Vr(3);
    wxr = B32Vr(4); wyr = B32Vr(5); wzr = B32Vr(6);
    
    axr = B32dVr(1); ayr = B32dVr(2); azr = B32dVr(3);
    dwxr = B32dVr(4); dwyr = B32dVr(5); dwzr = B32dVr(6);
    
    wx = B32V(4); wy = B32V(5); wz = B32V(6);
    
    B32g = B32_Rot_W*gravity.Wg;
    
    gx = B32g(1); gy = B32g(2); gz = B32g(3);
    
    Y11 = (-vyr * wz + vzr * wy + axr + gx);
    t5 = (wy * wyr);
    t6 = (wz * wzr);
    Y12 = -t5 - t6;
    t7 = (wxr * wy);
    Y13 = (t7 - dwzr);
    t8 = (wxr * wz);
    Y14  = (t8 + dwyr);
    Y15 = 0;
    Y16 = 0;
    Y17 = 0;
    Y18  = 0;
    Y19 = 0;
    Y110 = 0;
    Y111 = 0;
    Y112 = 0;
    Y113 = 0;
    Y21 = vxr * wz - vzr * wx + ayr + gy;
    t11 = wx * wyr;
    Y22 = t11 + dwzr;
    t12 = wx * wxr;
    Y23 = -t12 - t6;
    t13 = wyr * wz;
    Y24 = t13 - dwxr;
    Y25 = 0;
    Y26 = 0;
    Y27 = 0;
    Y28 = 0;
    Y29 = 0;
    Y210 = 0;
    Y211 = 0;
    Y212 = 0;
    Y213 = 0;
    Y31 = -vxr * wy + vyr * wx + azr + gz;
    t16 = wx * wzr;
    Y32 = t16 - dwyr;
    t17 = wy * wzr;
    Y33 = t17 + dwxr;
    Y34 = -t12 - t5;
    Y35 = 0;
    Y36 = 0;
    Y37 = 0;
    Y38 = 0;
    Y39 = 0;
    Y310 = 0;
    Y311 = 0;
    Y312 = 0;
    Y313 = 0;
    Y41 = 0;
    Y42 = 0;
    Y43 = Y31;
    Y44 = -Y21;
    Y45 = 0;
    Y46 = Y33;
    Y47 = -Y24;
    Y48 = Y32;
    Y49 = -Y22;
    Y410 = -t5 + t6;
    Y411 = t17 - t13 + dwxr;
    Y412 = -t13;
    Y413 = t17;
    Y51 = 0;
    Y52 = -Y43;
    Y53 = 0;
    Y54 = Y11;
    Y55 = -Y48;
    Y56 = 0;
    Y57 = Y14;
    Y58 = -Y46;
    Y59 = t12 - t6;
    Y510 = Y13;
    Y511 = t8;
    Y512 = -t16 + Y511 + dwyr;
    Y513 = -t16;
    Y61 = 0;
    Y62 = Y21;
    Y63 = -Y54;
    Y64 = 0;
    Y65 = Y22;
    Y66 = -Y510;
    Y67 = 0;
    Y68 = -t12 + t5;
    Y69 = Y24;
    Y610 = -Y57;
    Y611 = -t7;
    Y612 = t11;
    Y613 = Y612 + Y611 + dwzr;
    
    
    YB32r = [Y11 Y12 Y13 Y14 Y15 Y16 Y17 Y18 Y19 Y110 Y111 Y112 Y113;...
             Y21 Y22 Y23 Y24 Y25 Y26 Y27 Y28 Y29 Y210 Y211 Y212 Y213;...
             Y31 Y32 Y33 Y34 Y35 Y36 Y37 Y38 Y39 Y310 Y311 Y312 Y313;...
             Y41 Y42 Y43 Y44 Y45 Y46 Y47 Y48 Y49 Y410 Y411 Y412 Y413;...
             Y51 Y52 Y53 Y54 Y55 Y56 Y57 Y58 Y59 Y510 Y511 Y512 Y513;...
             Y61 Y62 Y63 Y64 Y65 Y66 Y67 Y68 Y69 Y610 Y611 Y612 Y613];

end

== matlab function VDCHyd2022a/sbVDCController/sbFormTotalRequiredForces/sbTotalRequiredForcesRS2/regressorYB42r ==
  data: B42Vr input; B42dVr input; B42V input; B42_Rot_W input; gravity parameter; YB42r output
function YB42r  = inertiaRegressor(B42Vr, B42dVr, B42V, B42_Rot_W,  gravity)

    % Forms regressor matrix YB42r as described in Appendix A of
    % Zhu, Wen-Hong. Virtual decomposition control: toward hyper degrees
    % of freedom robots. Vol. 60. Springer Science & Business Media, 2010.

    % The code below is not the most apparent 1-to-1 visual mapping to the
    % book equations since it was generated using a symbolic toolbox.

    vxr = B42Vr(1); vyr = B42Vr(2); vzr = B42Vr(3);
    wxr = B42Vr(4); wyr = B42Vr(5); wzr = B42Vr(6);
    
    axr = B42dVr(1); ayr = B42dVr(2); azr = B42dVr(3);
    dwxr = B42dVr(4); dwyr = B42dVr(5); dwzr = B42dVr(6);
    
    wx = B42V(4); wy = B42V(5); wz = B42V(6);
    
    B42g = B42_Rot_W*gravity.Wg;
    
    gx = B42g(1); gy = B42g(2); gz = B42g(3);
    
    Y11 = (-vyr * wz + vzr * wy + axr + gx);
    t5 = (wy * wyr);
    t6 = (wz * wzr);
    Y12 = -t5 - t6;
    t7 = (wxr * wy);
    Y13 = (t7 - dwzr);
    t8 = (wxr * wz);
    Y14  = (t8 + dwyr);
    Y15 = 0;
    Y16 = 0;
    Y17 = 0;
    Y18  = 0;
    Y19 = 0;
    Y110 = 0;
    Y111 = 0;
    Y112 = 0;
    Y113 = 0;
    Y21 = vxr * wz - vzr * wx + ayr + gy;
    t11 = wx * wyr;
    Y22 = t11 + dwzr;
    t12 = wx * wxr;
    Y23 = -t12 - t6;
    t13 = wyr * wz;
    Y24 = t13 - dwxr;
    Y25 = 0;
    Y26 = 0;
    Y27 = 0;
    Y28 = 0;
    Y29 = 0;
    Y210 = 0;
    Y211 = 0;
    Y212 = 0;
    Y213 = 0;
    Y31 = -vxr * wy + vyr * wx + azr + gz;
    t16 = wx * wzr;
    Y32 = t16 - dwyr;
    t17 = wy * wzr;
    Y33 = t17 + dwxr;
    Y34 = -t12 - t5;
    Y35 = 0;
    Y36 = 0;
    Y37 = 0;
    Y38 = 0;
    Y39 = 0;
    Y310 = 0;
    Y311 = 0;
    Y312 = 0;
    Y313 = 0;
    Y41 = 0;
    Y42 = 0;
    Y43 = Y31;
    Y44 = -Y21;
    Y45 = 0;
    Y46 = Y33;
    Y47 = -Y24;
    Y48 = Y32;
    Y49 = -Y22;
    Y410 = -t5 + t6;
    Y411 = t17 - t13 + dwxr;
    Y412 = -t13;
    Y413 = t17;
    Y51 = 0;
    Y52 = -Y43;
    Y53 = 0;
    Y54 = Y11;
    Y55 = -Y48;
    Y56 = 0;
    Y57 = Y14;
    Y58 = -Y46;
    Y59 = t12 - t6;
    Y510 = Y13;
    Y511 = t8;
    Y512 = -t16 + Y511 + dwyr;
    Y513 = -t16;
    Y61 = 0;
    Y62 = Y21;
    Y63 = -Y54;
    Y64 = 0;
    Y65 = Y22;
    Y66 = -Y510;
    Y67 = 0;
    Y68 = -t12 + t5;
    Y69 = Y24;
    Y610 = -Y57;
    Y611 = -t7;
    Y612 = t11;
    Y613 = Y612 + Y611 + dwzr;
    
    
    YB42r = [Y11 Y12 Y13 Y14 Y15 Y16 Y17 Y18 Y19 Y110 Y111 Y112 Y113;...
             Y21 Y22 Y23 Y24 Y25 Y26 Y27 Y28 Y29 Y210 Y211 Y212 Y213;...
             Y31 Y32 Y33 Y34 Y35 Y36 Y37 Y38 Y39 Y310 Y311 Y312 Y313;...
             Y41 Y42 Y43 Y44 Y45 Y46 Y47 Y48 Y49 Y410 Y411 Y412 Y413;...
             Y51 Y52 Y53 Y54 Y55 Y56 Y57 Y58 Y59 Y510 Y511 Y512 Y513;...
             Y61 Y62 Y63 Y64 Y65 Y66 Y67 Y68 Y69 Y610 Y611 Y612 Y613];

end

== matlab function VDCHyd2022a/sbVDCController/sbFormTotalRequiredForces/sbTotalRequiredForcesRS2/regressorYBc2r ==
  data: Bc2Vr input; Bc2dVr input; Bc2V input; Bc2_Rot_W input; gravity parameter; YBc2r output
function YBc2r  = inertiaRegressor(Bc2Vr, Bc2dVr, Bc2V, Bc2_Rot_W,  gravity)

    % Forms regressor matrix YBc2r as described in Appendix A of
    % Zhu, Wen-Hong. Virtual decomposition control: toward hyper degrees
    % of freedom robots. Vol. 60. Springer Science & Business Media, 2010.

    % The code below is not the most apparent 1-to-1 visual mapping to the
    % book equations since it was generated using a symbolic toolbox.

    vxr = Bc2Vr(1); vyr = Bc2Vr(2); vzr = Bc2Vr(3);
    wxr = Bc2Vr(4); wyr = Bc2Vr(5); wzr = Bc2Vr(6);
    
    axr = Bc2dVr(1); ayr = Bc2dVr(2); azr = Bc2dVr(3);
    dwxr = Bc2dVr(4); dwyr = Bc2dVr(5); dwzr = Bc2dVr(6);
    
    wx = Bc2V(4); wy = Bc2V(5); wz = Bc2V(6);
    
    Bc2g = Bc2_Rot_W*gravity.Wg;
    
    gx = Bc2g(1); gy = Bc2g(2); gz = Bc2g(3);
    
    Y11 = (-vyr * wz + vzr * wy + axr + gx);
    t5 = (wy * wyr);
    t6 = (wz * wzr);
    Y12 = -t5 - t6;
    t7 = (wxr * wy);
    Y13 = (t7 - dwzr);
    t8 = (wxr * wz);
    Y14  = (t8 + dwyr);
    Y15 = 0;
    Y16 = 0;
    Y17 = 0;
    Y18  = 0;
    Y19 = 0;
    Y110 = 0;
    Y111 = 0;
    Y112 = 0;
    Y113 = 0;
    Y21 = vxr * wz - vzr * wx + ayr + gy;
    t11 = wx * wyr;
    Y22 = t11 + dwzr;
    t12 = wx * wxr;
    Y23 = -t12 - t6;
    t13 = wyr * wz;
    Y24 = t13 - dwxr;
    Y25 = 0;
    Y26 = 0;
    Y27 = 0;
    Y28 = 0;
    Y29 = 0;
    Y210 = 0;
    Y211 = 0;
    Y212 = 0;
    Y213 = 0;
    Y31 = -vxr * wy + vyr * wx + azr + gz;
    t16 = wx * wzr;
    Y32 = t16 - dwyr;
    t17 = wy * wzr;
    Y33 = t17 + dwxr;
    Y34 = -t12 - t5;
    Y35 = 0;
    Y36 = 0;
    Y37 = 0;
    Y38 = 0;
    Y39 = 0;
    Y310 = 0;
    Y311 = 0;
    Y312 = 0;
    Y313 = 0;
    Y41 = 0;
    Y42 = 0;
    Y43 = Y31;
    Y44 = -Y21;
    Y45 = 0;
    Y46 = Y33;
    Y47 = -Y24;
    Y48 = Y32;
    Y49 = -Y22;
    Y410 = -t5 + t6;
    Y411 = t17 - t13 + dwxr;
    Y412 = -t13;
    Y413 = t17;
    Y51 = 0;
    Y52 = -Y43;
    Y53 = 0;
    Y54 = Y11;
    Y55 = -Y48;
    Y56 = 0;
    Y57 = Y14;
    Y58 = -Y46;
    Y59 = t12 - t6;
    Y510 = Y13;
    Y511 = t8;
    Y512 = -t16 + Y511 + dwyr;
    Y513 = -t16;
    Y61 = 0;
    Y62 = Y21;
    Y63 = -Y54;
    Y64 = 0;
    Y65 = Y22;
    Y66 = -Y510;
    Y67 = 0;
    Y68 = -t12 + t5;
    Y69 = Y24;
    Y610 = -Y57;
    Y611 = -t7;
    Y612 = t11;
    Y613 = Y612 + Y611 + dwzr;
    
    
    YBc2r = [Y11 Y12 Y13 Y14 Y15 Y16 Y17 Y18 Y19 Y110 Y111 Y112 Y113;...
             Y21 Y22 Y23 Y24 Y25 Y26 Y27 Y28 Y29 Y210 Y211 Y212 Y213;...
             Y31 Y32 Y33 Y34 Y35 Y36 Y37 Y38 Y39 Y310 Y311 Y312 Y313;...
             Y41 Y42 Y43 Y44 Y45 Y46 Y47 Y48 Y49 Y410 Y411 Y412 Y413;...
             Y51 Y52 Y53 Y54 Y55 Y56 Y57 Y58 Y59 Y510 Y511 Y512 Y513;...
             Y61 Y62 Y63 Y64 Y65 Y66 Y67 Y68 Y69 Y610 Y611 Y612 Y613];

end

== matlab function VDCHyd2022a/sbVDCController/sbFormingControlActions/controlVoltagePS2 ==
  data: uft2r input; pS input; pR input; pat2 input; pbt2 input; xt2 input; ut2 output; thetavt2 input; hosingT2 parameter; cylT2 parameter
function ut2  = calculateControlVoltage(uft2r, pS, pR, pat2, pbt2, xt2, thetavt2, hosingT2, cylT2)

    cp1 = thetavt2(1); cn1=thetavt2(2); cp2=thetavt2(3); cn2=thetavt2(4);

    % Implemented per (27) in S. Lampinen, J. Koivumäki and J. Mattila, 
    % "Improved Hydraulic Cylinder Model for the Virtual Decomposition 
    % Control Approach," 2019 IEEE International Conference on Cybernetics 
    % and Intelligent Systems (CIS) and IEEE Conference on Robotics, 
    % Automation and Mechatronics (RAM), Bangkok, Thailand, 2019, 
    % pp. 113-118, doi: 10.1109/CIS-RAM47153.2019.9095788 
    ut2 = uft2r*selFcn(uft2r)/( (cp1*sqAbsPresDrop(pS-pat2))/(hosingT2.V0a/cylT2.Aa + xt2) + (cn2*sqAbsPresDrop(pbt2-pR))/(hosingT2.V0b/cylT2.Ab + cylT2.sp - xt2) ) + ...
          uft2r*selFcn(-uft2r)/( (cp2*sqAbsPresDrop(pS-pbt2))/(hosingT2.V0b/cylT2.Ab + cylT2.sp - xt2) + (cn1*sqAbsPresDrop(pat2-pR))/(hosingT2.V0a/cylT2.Aa + xt2) );


end


function S = selFcn(U)

    if U > 0
        S = 1;
    else
        S = 0;
    end
    
end

function nup = sqAbsPresDrop(dp)

    nup = sign(dp)*sqrt(abs(dp));

end

== matlab function VDCHyd2022a/sbVDCController/sbFormTotalRequiredForces/sbTotalRequiredForcesRS1/regressorYB11r ==
  data: B11Vr input; B11dVr input; B11V input; B11_Rot_W input; gravity parameter; YB11r output
function YB11r  = inertiaRegressor(B11Vr, B11dVr, B11V, B11_Rot_W,  gravity)

    % Forms regressor matrix YB11r as described in Appendix A of
    % Zhu, Wen-Hong. Virtual decomposition control: toward hyper degrees
    % of freedom robots. Vol. 60. Springer Science & Business Media, 2010.

    % The code below is not the most apparent 1-to-1 visual mapping to the
    % book equations since it was generated using a symbolic toolbox.
    
    vxr = B11Vr(1); vyr = B11Vr(2); vzr = B11Vr(3);
    wxr = B11Vr(4); wyr = B11Vr(5); wzr = B11Vr(6);
    
    axr = B11dVr(1); ayr = B11dVr(2); azr = B11dVr(3);
    dwxr = B11dVr(4); dwyr = B11dVr(5); dwzr = B11dVr(6);
    
    wx = B11V(4); wy = B11V(5); wz = B11V(6);
    
    B11g = B11_Rot_W*gravity.Wg;
    
    gx = B11g(1); gy = B11g(2); gz = B11g(3);
    
    Y11 = (-vyr * wz + vzr * wy + axr + gx);
    t5 = (wy * wyr);
    t6 = (wz * wzr);
    Y12 = -t5 - t6;
    t7 = (wxr * wy);
    Y13 = (t7 - dwzr);
    t8 = (wxr * wz);
    Y14  = (t8 + dwyr);
    Y15 = 0;
    Y16 = 0;
    Y17 = 0;
    Y18  = 0;
    Y19 = 0;
    Y110 = 0;
    Y111 = 0;
    Y112 = 0;
    Y113 = 0;
    Y21 = vxr * wz - vzr * wx + ayr + gy;
    t11 = wx * wyr;
    Y22 = t11 + dwzr;
    t12 = wx * wxr;
    Y23 = -t12 - t6;
    t13 = wyr * wz;
    Y24 = t13 - dwxr;
    Y25 = 0;
    Y26 = 0;
    Y27 = 0;
    Y28 = 0;
    Y29 = 0;
    Y210 = 0;
    Y211 = 0;
    Y212 = 0;
    Y213 = 0;
    Y31 = -vxr * wy + vyr * wx + azr + gz;
    t16 = wx * wzr;
    Y32 = t16 - dwyr;
    t17 = wy * wzr;
    Y33 = t17 + dwxr;
    Y34 = -t12 - t5;
    Y35 = 0;
    Y36 = 0;
    Y37 = 0;
    Y38 = 0;
    Y39 = 0;
    Y310 = 0;
    Y311 = 0;
    Y312 = 0;
    Y313 = 0;
    Y41 = 0;
    Y42 = 0;
    Y43 = Y31;
    Y44 = -Y21;
    Y45 = 0;
    Y46 = Y33;
    Y47 = -Y24;
    Y48 = Y32;
    Y49 = -Y22;
    Y410 = -t5 + t6;
    Y411 = t17 - t13 + dwxr;
    Y412 = -t13;
    Y413 = t17;
    Y51 = 0;
    Y52 = -Y43;
    Y53 = 0;
    Y54 = Y11;
    Y55 = -Y48;
    Y56 = 0;
    Y57 = Y14;
    Y58 = -Y46;
    Y59 = t12 - t6;
    Y510 = Y13;
    Y511 = t8;
    Y512 = -t16 + Y511 + dwyr;
    Y513 = -t16;
    Y61 = 0;
    Y62 = Y21;
    Y63 = -Y54;
    Y64 = 0;
    Y65 = Y22;
    Y66 = -Y510;
    Y67 = 0;
    Y68 = -t12 + t5;
    Y69 = Y24;
    Y610 = -Y57;
    Y611 = -t7;
    Y612 = t11;
    Y613 = Y612 + Y611 + dwzr;
    
    
    YB11r = [Y11 Y12 Y13 Y14 Y15 Y16 Y17 Y18 Y19 Y110 Y111 Y112 Y113;...
             Y21 Y22 Y23 Y24 Y25 Y26 Y27 Y28 Y29 Y210 Y211 Y212 Y213;...
             Y31 Y32 Y33 Y34 Y35 Y36 Y37 Y38 Y39 Y310 Y311 Y312 Y313;...
             Y41 Y42 Y43 Y44 Y45 Y46 Y47 Y48 Y49 Y410 Y411 Y412 Y413;...
             Y51 Y52 Y53 Y54 Y55 Y56 Y57 Y58 Y59 Y510 Y511 Y512 Y513;...
             Y61 Y62 Y63 Y64 Y65 Y66 Y67 Y68 Y69 Y610 Y611 Y612 Y613];

end

== matlab function VDCHyd2022a/sbVDCController/sbFormTotalRequiredForces/sbTotalRequiredForcesRS1/regressorYB31r ==
  data: B31Vr input; B31dVr input; B31V input; B31_Rot_W input; gravity parameter; YB31r output
function YB31r  = inertiaRegressor(B31Vr, B31dVr, B31V, B31_Rot_W,  gravity)

    % Forms regressor matrix YB31r as described in Appendix A of
    % Zhu, Wen-Hong. Virtual decomposition control: toward hyper degrees
    % of freedom robots. Vol. 60. Springer Science & Business Media, 2010.

    % The code below is not the most apparent 1-to-1 visual mapping to the
    % book equations since it was generated using a symbolic toolbox.

    vxr = B31Vr(1); vyr = B31Vr(2); vzr = B31Vr(3);
    wxr = B31Vr(4); wyr = B31Vr(5); wzr = B31Vr(6);
    
    axr = B31dVr(1); ayr = B31dVr(2); azr = B31dVr(3);
    dwxr = B31dVr(4); dwyr = B31dVr(5); dwzr = B31dVr(6); 
    
    wx = B31V(4); wy = B31V(5); wz = B31V(6);
    
    B31g = B31_Rot_W*gravity.Wg;
    
    gx = B31g(1); gy = B31g(2); gz = B31g(3);
    
    Y11 = (-vyr * wz + vzr * wy + axr + gx);
    t5 = (wy * wyr);
    t6 = (wz * wzr);
    Y12 = -t5 - t6;
    t7 = (wxr * wy);
    Y13 = (t7 - dwzr);
    t8 = (wxr * wz);
    Y14  = (t8 + dwyr);
    Y15 = 0;
    Y16 = 0;
    Y17 = 0;
    Y18  = 0;
    Y19 = 0;
    Y110 = 0;
    Y111 = 0;
    Y112 = 0;
    Y113 = 0;
    Y21 = vxr * wz - vzr * wx + ayr + gy;
    t11 = wx * wyr;
    Y22 = t11 + dwzr;
    t12 = wx * wxr;
    Y23 = -t12 - t6;
    t13 = wyr * wz;
    Y24 = t13 - dwxr;
    Y25 = 0;
    Y26 = 0;
    Y27 = 0;
    Y28 = 0;
    Y29 = 0;
    Y210 = 0;
    Y211 = 0;
    Y212 = 0;
    Y213 = 0;
    Y31 = -vxr * wy + vyr * wx + azr + gz;
    t16 = wx * wzr;
    Y32 = t16 - dwyr;
    t17 = wy * wzr;
    Y33 = t17 + dwxr;
    Y34 = -t12 - t5;
    Y35 = 0;
    Y36 = 0;
    Y37 = 0;
    Y38 = 0;
    Y39 = 0;
    Y310 = 0;
    Y311 = 0;
    Y312 = 0;
    Y313 = 0;
    Y41 = 0;
    Y42 = 0;
    Y43 = Y31;
    Y44 = -Y21;
    Y45 = 0;
    Y46 = Y33;
    Y47 = -Y24;
    Y48 = Y32;
    Y49 = -Y22;
    Y410 = -t5 + t6;
    Y411 = t17 - t13 + dwxr;
    Y412 = -t13;
    Y413 = t17;
    Y51 = 0;
    Y52 = -Y43;
    Y53 = 0;
    Y54 = Y11;
    Y55 = -Y48;
    Y56 = 0;
    Y57 = Y14;
    Y58 = -Y46;
    Y59 = t12 - t6;
    Y510 = Y13;
    Y511 = t8;
    Y512 = -t16 + Y511 + dwyr;
    Y513 = -t16;
    Y61 = 0;
    Y62 = Y21;
    Y63 = -Y54;
    Y64 = 0;
    Y65 = Y22;
    Y66 = -Y510;
    Y67 = 0;
    Y68 = -t12 + t5;
    Y69 = Y24;
    Y610 = -Y57;
    Y611 = -t7;
    Y612 = t11;
    Y613 = Y612 + Y611 + dwzr;
    
    
    YB31r = [Y11 Y12 Y13 Y14 Y15 Y16 Y17 Y18 Y19 Y110 Y111 Y112 Y113;...
             Y21 Y22 Y23 Y24 Y25 Y26 Y27 Y28 Y29 Y210 Y211 Y212 Y213;...
             Y31 Y32 Y33 Y34 Y35 Y36 Y37 Y38 Y39 Y310 Y311 Y312 Y313;...
             Y41 Y42 Y43 Y44 Y45 Y46 Y47 Y48 Y49 Y410 Y411 Y412 Y413;...
             Y51 Y52 Y53 Y54 Y55 Y56 Y57 Y58 Y59 Y510 Y511 Y512 Y513;...
             Y61 Y62 Y63 Y64 Y65 Y66 Y67 Y68 Y69 Y610 Y611 Y612 Y613];

end
